simulink model "fec_prototype_02"  (R2013a)
settings: Solver=ode45  StartTime=0.0  StopTime=50  FixedStep=1  RelTol=1e-3
undefined symbols (not defined in the file or in its folder): EbNo, rsgenpoly
libraries: commutil2 x4, commdigbbndpm3 x2, commcnvcod2 x2, commblkintrlv2 x2, commblkcod2 x2, commrandsrc2 x1, dspquant2 x1, commchan3 x1, commsink2 x1
settings Model: Creator=lifesatrip  LastModifiedBy=lifesatrip

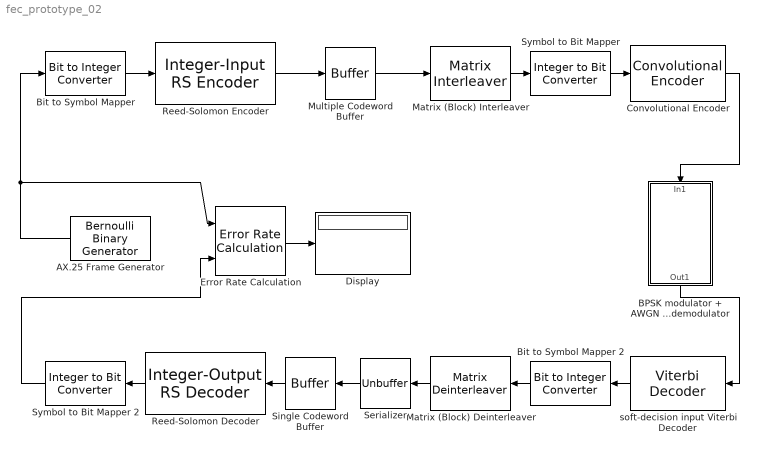
== system fec_prototype_02 ==
  "AX.25 Frame Generator " : commrandsrc2/Bernoulli Binary Generator  P=0.5  seed=61  Ts=1  frameBased=on  sampPerFrame=2  orient=off  outDataType=double
  BPSK modulator + AWGN w/ bursty noise + soft-decision BPSK demodulator : Subsystem
  Bit to Symbol Mapper : commutil2/Bit to Integer Converter  nbits=2  bitOrder=MSB first  signedOutputValues=Unsigned  outDtype=double  outDtypeSigned=Inherit via internal rule
  Bit to Symbol Mapper 2 : commutil2/Bit to Integer Converter  nbits=2  bitOrder=MSB first  signedOutputValues=Unsigned  outDtype=double  outDtypeSigned=Inherit via internal rule
  Convolutional Encoder : commcnvcod2/Convolutional Encoder  trellis=poly2trellis(9, [561 753])  opMode=Continuous  DelayedResetAction=off  hasIniStPort=off  hasFinStPort=off  usePuncVector=off  punctureVector=[1 1 0 1 1 0].'  reset=Unused parameter value
  Display : Display
  Error Rate Calculation : commsink2/Error Rate Calculation  N=15  st_delay=0  cp_mode=Entire frame  subframe=[]  PMode=Port  WsName=ErrorVec  RsMode2=off  stop=off  numErr=100  maxBits=1e6
  Matrix (Block) Deinterleaver : commblkintrlv2/Matrix Deinterleaver  Nrows=3  Ncols=7
  Matrix (Block) Interleaver : commblkintrlv2/Matrix Interleaver  Nrows=3  Ncols=7
  Multiple Codeword Buffer : Buffer  N=21  TreatMby1Signals=One channel
  Reed-Solomon Decoder : commblkcod2/Integer-Output RS Decoder  n=7  k=1  specPrimPoly=off  prPoly=[1 0 1 1]  specGenPoly=off  genPoly=rsgenpoly(7,3)  specPuncture=off  punctVec=[ones(2,1); zeros(2,1)]  specErasurePort=off  showNumErr=off
  "Reed-Solomon Encoder " : commblkcod2/Integer-Input RS Encoder  n=7  k=1  specPrimPoly=off  prPoly=[1 0 1 1]  specGenPoly=off  genPoly=rsgenpoly(7,3)  specPuncture=off  punctVec=[ones(2,1); zeros(2,1)]
  Serializer : Unbuffer  SampleBasedProcessing=Same as frame based
  Single Codeword Buffer : Buffer  N=7  TreatMby1Signals=One channel
  Symbol to Bit Mapper 2 : commutil2/Integer to Bit Converter  nbits=2  signedInputValues=Unsigned  bitOrder=MSB first  outDtype=Inherit via internal rule
  Symbol to Bit Mapper : commutil2/Integer to Bit Converter  nbits=2  signedInputValues=Unsigned  bitOrder=MSB first  outDtype=boolean
  soft-decision input Viterbi Decoder : commcnvcod2/Viterbi Decoder  trellis=poly2trellis(9, [561 753])  isPunctured=off  punctureVector=[1 1 0 1 1 0].'  erasures=off  dectype=Soft decision  runSigValErrCheck=off  nsdecb=3  smWordLength=6  tbdepth=6  opmode=Continuous  reset=off  outDataType=boolean  delayedResetAction=off
  wires:
  Error Rate Calculation/1 -> Display/1
  "AX.25 Frame Generator "/1 -> Bit to Symbol Mapper/1, Error Rate Calculation/1
  Matrix (Block) Interleaver/1 -> Symbol to Bit Mapper/1
  Symbol to Bit Mapper/1 -> Convolutional Encoder/1
  Multiple Codeword Buffer/1 -> Matrix (Block) Interleaver/1
  soft-decision input Viterbi Decoder/1 -> Bit to Symbol Mapper 2/1
  Bit to Symbol Mapper 2/1 -> Matrix (Block) Deinterleaver/1
  Matrix (Block) Deinterleaver/1 -> Serializer/1
  Serializer/1 -> Single Codeword Buffer/1
  Single Codeword Buffer/1 -> Reed-Solomon Decoder/1
  Reed-Solomon Decoder/1 -> Symbol to Bit Mapper 2/1
  "Reed-Solomon Encoder "/1 -> Multiple Codeword Buffer/1
  Symbol to Bit Mapper 2/1 -> Error Rate Calculation/2
  Bit to Symbol Mapper/1 -> "Reed-Solomon Encoder "/1
  Convolutional Encoder/1 -> BPSK modulator + AWGN w/ bursty noise + soft-decision BPSK demodulator/1(In1)
  BPSK modulator + AWGN w/ bursty noise + soft-decision BPSK demodulator/1(Out1) -> soft-decision input Viterbi Decoder/1

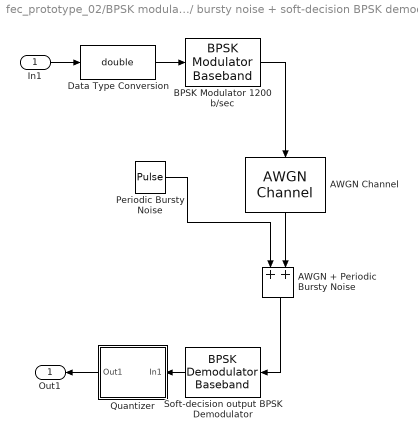
== system fec_prototype_02/BPSK modulator + AWGN w// bursty noise + soft-decision BPSK demodulator ==
  In1 : Inport
  " Quantizer" : Subsystem
  AWGN Channel : commchan3/AWGN Channel  InputProcessing=Columns as channels (frame based)  seed=113  noiseMode="Signal to noise ratio  (Eb/No)"  EbNodB=EbNo - 10*log10(2)  EsNodB=1  SNRdB=10  bitsPerSym=1  Ps=1  Tsym=1  variance=(1*0.005)/((1/200)*10^(EbNo/10))
  AWGN + Periodic Bursty Noise : Sum
  BPSK Modulator 1200 b/sec : commdigbbndpm3/BPSK Modulator Baseband  Ph=0  outDtype=double  outWordLen=16  outUDDataType=sfix(16)  outFracLenMode=Best precision  outFracLen=15
  Data Type Conversion : DataTypeConversion  OutDataTypeStr=double
  "Periodic Bursty Noise " : DiscretePulseGenerator  PulseType=Time based  Period=10  PulseWidth=5
  "Soft-decision output BPSK Demodulator " : commdigbbndpm3/BPSK Demodulator Baseband  Ph=0  DecType=Log-likelihood ratio  VarSource=Dialog  Variance=1/(10^((EbNo-10*log10(2))/10))  outDtype=double  derotateFactorWordLen=16
  Out1 : Outport
  wires:
  AWGN + Periodic Bursty Noise/1 -> "Soft-decision output BPSK Demodulator "/1
  AWGN Channel/1 -> AWGN + Periodic Bursty Noise/2
  "Periodic Bursty Noise "/1 -> AWGN + Periodic Bursty Noise/1
  BPSK Modulator 1200 b/sec/1 -> AWGN Channel/1
  Data Type Conversion/1 -> BPSK Modulator 1200 b/sec/1
  "Soft-decision output BPSK Demodulator "/1 -> " Quantizer"/1(In1)
  In1/1 -> Data Type Conversion/1
  " Quantizer"/1(Out1) -> Out1/1

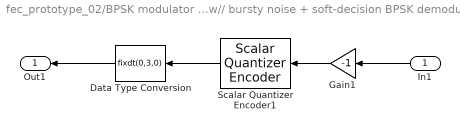
== system fec_prototype_02/BPSK modulator + AWGN w// bursty noise + soft-decision BPSK demodulator/ Quantizer ==
  In1 : Inport
  Data Type Conversion : DataTypeConversion  OutDataTypeStr=fixdt(0,3,0)
  Gain1 : Gain  Gain=-1
  Scalar Quantizer Encoder1 : dspquant2/Scalar Quantizer Encoder  paramSrc=Specify via dialog  partType=Unbounded  BBoundary=[-6:2:6]/4  UBoundary=[-3:3]  SearchMethod=Linear  tieBreakRule=Choose the higher index  outQU=off  outQError=off  codebook=[1.5:9.5]  outStatus=off  invalidin=Clip  idtype=uint8  roundingMode=Floor  overflowMode=off
  Out1 : Outport
  wires:
  In1/1 -> Gain1/1
  Data Type Conversion/1 -> Out1/1
  Scalar Quantizer Encoder1/1 -> Data Type Conversion/1
  Gain1/1 -> Scalar Quantizer Encoder1/1
